simulink model "item4ModeloNLin"  (R2018a)
settings: Solver=VariableStepAuto  StartTime=0.0  StopTime=50  RelTol=1e-3
libraries: simulink x2
settings Model: Creator=julia  LastModifiedBy=crist
settings CodeAppCC: StateflowObjectComments=on

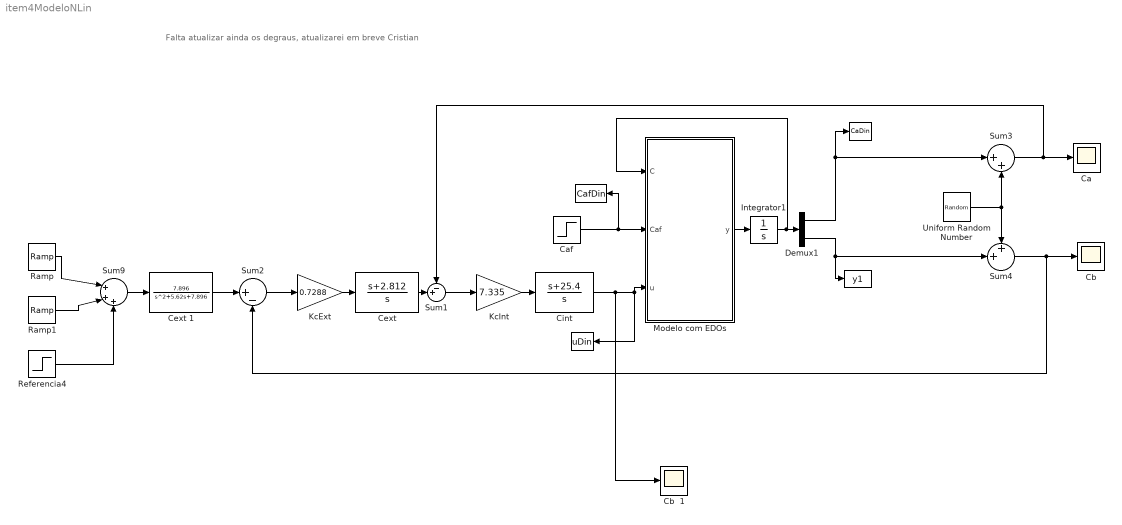
== system item4ModeloNLin ==
  note: Falta atualizar ainda os degraus, atualizarei em breve Cristian
  "   " : ToWorkspace  VariableName=y1  SaveFormat=Timeseries  SampleTime=-1
  "          " : ToWorkspace  VariableName=CafDin  SaveFormat=Timeseries  SampleTime=-1
  "                 " : ToWorkspace  VariableName=uDin  SaveFormat=Timeseries  SampleTime=-1
  "                   " : ToWorkspace  VariableName=CaDin  SaveFormat=Timeseries  SampleTime=-1
  "Ca  " : Scope
  Caf : Step  Time=35  Before=5.1  After=5.15  SampleTime=0
  "Cb  " : Scope
  Cb  1 : Scope
  "Cext " : TransferFcn  Numerator=[1 2.812]  Denominator=[1 0]
  Cext 1 : TransferFcn  Numerator=[7.896]  Denominator=[1 5.62 7.896]
  Cint : TransferFcn  Numerator=[1 25.4]  Denominator=[1 0]
  Demux1 : Demux  Outputs=2
  Integrator1 : Integrator  InitialCondition=[0;0]
  "KcExt " : Gain  Gain=0.7288
  "KcInt " : Gain  Gain=7.335
  Modelo com EDOs : MATLAB Function  TreatAsAtomicUnit=on
  Ramp : simulink/Sources/Ramp  slope=2.345/10  start=0  InitialOutput=0
  Ramp1 : simulink/Sources/Ramp  slope=-2.345/10  start=10  InitialOutput=0
  Referencia4 : Step  Time=20  After=0.25  SampleTime=0
  Sum1 : Sum  Inputs=-+|
  Sum2 : Sum  Inputs=|+-
  Sum3 : Sum  Inputs=|++
  Sum4 : Sum  Inputs=++|
  Sum9 : Sum  Inputs=|+++
  Uniform Random Number : UniformRandomNumber  Minimum=-0.005  Maximum=0.005  SampleTime=0.1
  wires:
  Modelo com EDOs/1(y) -> Integrator1/1
  Integrator1/1 -> Modelo com EDOs/1(C), Demux1/1
  Cint/1 -> Cb  1/1, Modelo com EDOs/3(u), "                 "/1
  Demux1/1 -> "                   "/1, Sum3/1
  Demux1/2 -> Sum4/2, "   "/1
  Caf/1 -> "          "/1, Modelo com EDOs/2(Caf)
  Referencia4/1 -> Sum9/3
  Ramp1/1 -> Sum9/2
  Ramp/1 -> Sum9/1
  "KcInt "/1 -> Cint/1
  Sum1/1 -> "KcInt "/1
  Sum2/1 -> "KcExt "/1
  "KcExt "/1 -> "Cext "/1
  "Cext "/1 -> Sum1/2
  Sum3/1 -> Sum1/1, "Ca  "/1
  Sum4/1 -> Sum2/2, "Cb  "/1
  Uniform Random Number/1 -> Sum3/2, Sum4/1
  Sum9/1 -> Cext 1/1
  Cext 1/1 -> Sum2/1

== matlab function item4ModeloNLin/Modelo com EDOs ==
  data: y output; C input; Caf input; u input
%EDOs das concentracoes dos produtos A e B
function y = fcn(C, Caf, u)

%constantes
k1 = 6.01; %L/min
k2 = 0.8433; %L/min
k3 = 0.1123; %mol/Lmin

%variaveis das concentracoes dos produtos A e B
Ca = C(1);
Cb = C(2);

%EDOs
Ca_d = -k1*Ca - k3*(Ca^2) + (Caf - Ca)*u;
Cb_d =  k1*Ca - k2*Cb - Cb*u;
 
%conjunto das EDOs
y = [Ca_d;Cb_d];
